simulink model "fuzzy_PI"  (R2015a)
settings: Solver=ode3  StartTime=0.0  StopTime=10.0  FixedStep=Ts  RelTol=1e-3
values from neighbouring files (symbols this model uses):
  K = 0.028    [fuzzy_PI_gains.m]    (also in task1.m; task2.m = 11.7; task3.m = 0.032)
  Kd = a*Ke    (= 0.075)    [fuzzy_PI_gains.m]    (also in task1.m; task2.m = 0.001558; task3.m)
  Ke = 0.5    [fuzzy_PI_gains.m]    (also in task1.m; task2.m = -0.0038; task3.m)
  Ts = 0.01    [fuzzy_PI_gains.m]    (also in task1.m; task2.m; task3.m)
libraries: fuzblock x1
settings Model: Creator=chris  LastModifiedBy=chris

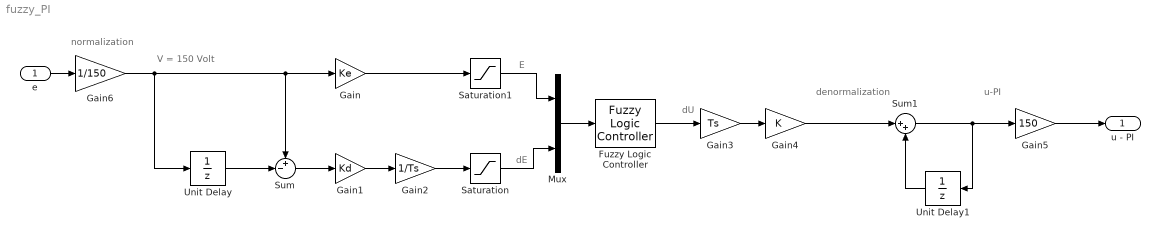
== system fuzzy_PI ==
  note: u-PI
  note: denormalization
  note: normalization
  note: dE
  note: E
  note: dU
  note: V = 150 Volt
  e : Inport
  Fuzzy Logic Controller : fuzblock/Fuzzy Logic  Controller  fis='myfis.fis'
  Gain : Gain  Gain=Ke
  Gain1 : Gain  Gain=Kd
  Gain2 : Gain  Gain=1/Ts
  Gain3 : Gain  Gain=Ts
  Gain4 : Gain  Gain=K
  Gain5 : Gain  Gain=150
  Gain6 : Gain  Gain=1/150
  Mux : Mux  Inputs=2
  Saturation : Saturate  UpperLimit=1  LowerLimit=-1
  Saturation1 : Saturate  UpperLimit=1  LowerLimit=-1
  Sum : Sum  Inputs=+-|
  Sum1 : Sum  Inputs=|++
  Unit Delay : UnitDelay  SampleTime=-1
  Unit Delay1 : UnitDelay  SampleTime=-1
  "u - PI " : Outport
  wires:
  e/1 -> Gain6/1
  Unit Delay/1 -> Sum/2
  Sum/1 -> Gain1/1
  Gain1/1 -> Gain2/1
  Gain2/1 -> Saturation/1
  Gain/1 -> Saturation1/1
  Saturation/1 -> Mux/2
  Saturation1/1 -> Mux/1
  Mux/1 -> Fuzzy Logic Controller/1
  Fuzzy Logic Controller/1 -> Gain3/1
  Gain3/1 -> Gain4/1
  Gain6/1 -> Gain/1, Sum/1, Unit Delay/1
  Gain4/1 -> Sum1/1
  Sum1/1 -> Gain5/1, Unit Delay1/1
  Unit Delay1/1 -> Sum1/2
  Gain5/1 -> "u - PI "/1
